simulink model "model_task1"  (R2022b)
settings: Solver=VariableStepAuto  StartTime=0.0  StopTime=10.0  RelTol=1e-3
undefined symbols (not defined in the file): A
settings Model: Creator=anton  LastModifiedBy=anton

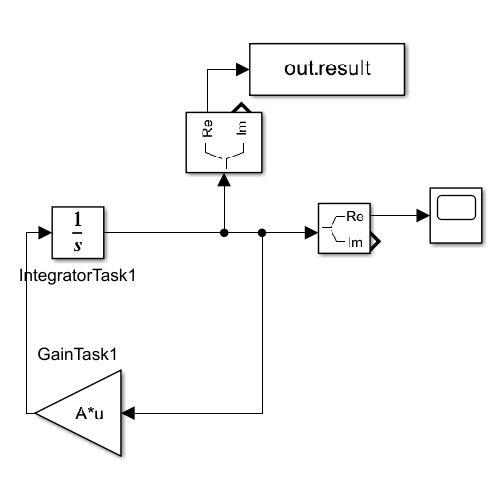
[thumbnail: Simulink's stored preview of the top-level diagram]
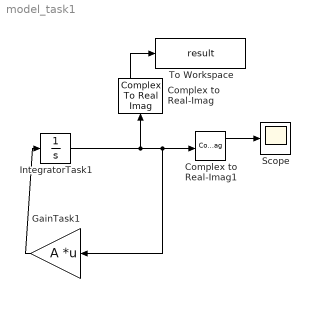
== system model_task1 ==
  Complex to Real-Imag : ComplexToRealImag
  Complex to Real-Imag1 : ComplexToRealImag
  GainTask1 : Gain  Gain=A  Multiplication=Matrix(K*u)  ParamDataTypeStr=double  OutDataTypeStr=double
  IntegratorTask1 : Integrator  InitialCondition=[-1;3]
  Scope : Scope
  To Workspace : ToWorkspace  VariableName=result  SaveFormat=Timeseries  SampleTime=-1
  wires:
  GainTask1/1 -> IntegratorTask1/1
  IntegratorTask1/1 -> Complex to Real-Imag/1, Complex to Real-Imag1/1, GainTask1/1
  Complex to Real-Imag1/1 -> Scope/1
  Complex to Real-Imag/1 -> To Workspace/1
